simulink model "Throtte_VehicleDynamicsModel"  (R2019b)
settings: Solver=VariableStepAuto  StartTime=0.0  StopTime=10.0  RelTol=1e-3
PreLoadFcn:
  | %initial condition
  | theta_eq = pi/6;
  | 
  | 
  | %parameters for throttle
  | J=2.54e-4;
  | Ks=0.2;
  | Kd=0.03;
  | theta_eq=pi/6;
  | Cs=0.3;
settings Model: Creator=spuny  LastModifiedBy=spuny
settings DebuggingCC: AlgebraicLoopMsg=none

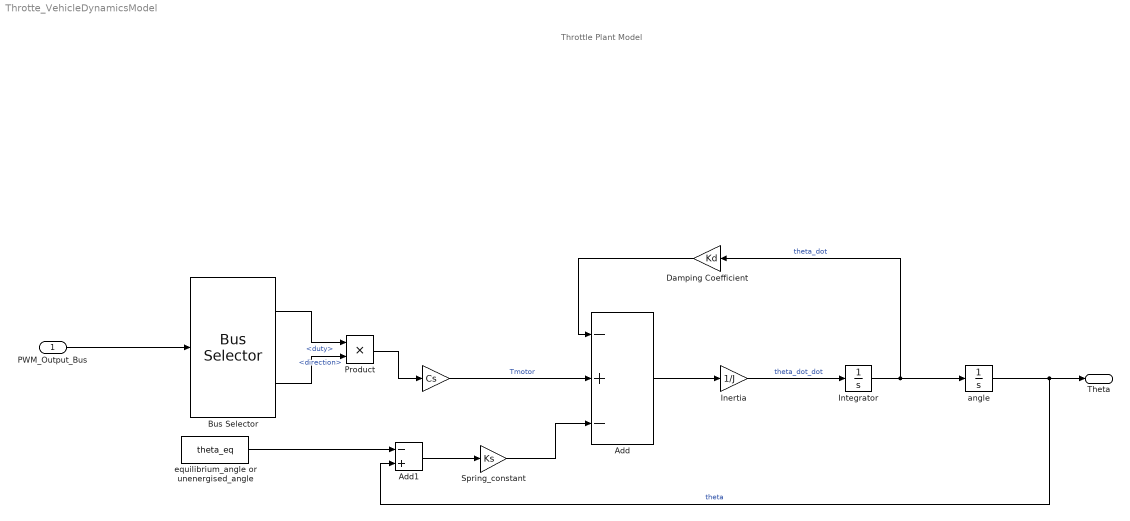
== system Throtte_VehicleDynamicsModel ==
  note: Throttle Plant Model
  "PWM_Output_Bus " : Inport  OutDataTypeStr=Bus: PWM_Output_Bus
  " " : Gain  Gain=Cs
  Add : Sum  Inputs=-+-
  Add1 : Sum  Inputs=-+
  Bus Selector : BusSelector  OutputSignals=duty,direction
  Damping Coefficient : Gain  Gain=Kd
  Inertia : Gain  Gain=1/J
  Integrator : Integrator
  Product : Product
  Spring_constant : Gain  Gain=Ks
  angle : Integrator  InitialCondition=pi/6  LimitOutput=on  UpperSaturationLimit=pi/2  LowerSaturationLimit=0
  equilibrium_angle or unenergised_angle : Constant  Value=theta_eq
  Theta : Outport
  wires:
  Product/1 -> " "/1
  " "/1 -> Add/2  "Tmotor"
  Add/1 -> Inertia/1
  Inertia/1 -> Integrator/1  "theta_dot_dot"
  Damping Coefficient/1 -> Add/1
  angle/1 -> Theta/1, Add1/2  "theta"
  equilibrium_angle or unenergised_angle/1 -> Add1/1
  Add1/1 -> Spring_constant/1
  Spring_constant/1 -> Add/3
  "PWM_Output_Bus "/1 -> Bus Selector/1
  Bus Selector/1 -> Product/1  "<duty>"
  Bus Selector/2 -> Product/2  "<direction>"
  Integrator/1 -> Damping Coefficient/1, angle/1  "theta_dot"
